simulink model "planta1"  (Simulink 7.3)
settings: Solver=ode45  StartTime=0.0  StopTime=240  RelTol=1e-3
settings Model: Creator=Luis Diaz  LastModifiedBy=gmujica

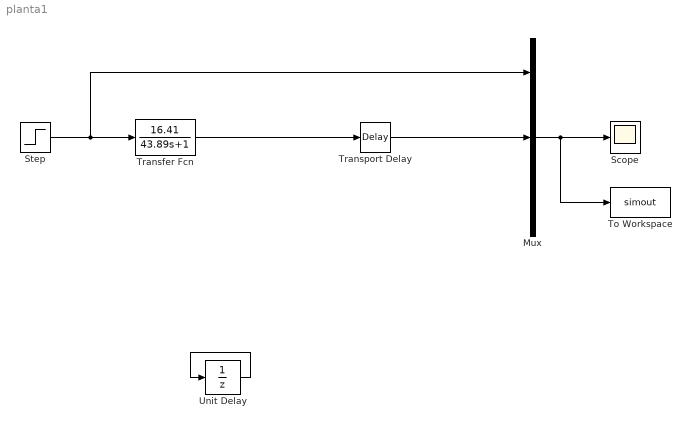
== system planta1 ==
  Mux : Mux  Inputs=3
  Scope : Scope
  Step : Step  Time=0.1  After=12  SampleTime=0
  To Workspace : ToWorkspace  VariableName=simout  SampleTime=-1  SaveFormat=Structure
  Transfer Fcn : TransferFcn  Numerator=[16.41]  Denominator=[43.89 1]
  Transport Delay : TransportDelay  DelayTime=0.5
  Unit Delay : UnitDelay  SampleTime=-1
  wires:
  Mux/1 -> Scope/1, To Workspace/1
  Step/1 -> Mux/1, Transfer Fcn/1
  Transfer Fcn/1 -> Transport Delay/1
  Transport Delay/1 -> Mux/2
  Unit Delay/1 -> Unit Delay/1
